simulink model "DataCenterStability"  (R2025b)
settings: Solver=daessc  StartTime=0  StopTime=7  FixedStep=5e-5  MaxStep=0.001  RelTol=1e-3
PostLoadFcn:
  | DataCenterParamScan
InitFcn:
  | opFile_ = fullfile(fileparts(which('DataCenterStability')), 'DataCenterStability_SteadyStateOP.mat');
  | if isfile(opFile_)
  |     tmp_ = load(opFile_, 'op');
  |     assignin('base', 'ssOP__', tmp_.op);
  | end
  | warning('off','physmod:common:mf:system:xform:DelayUnsupportedWithOperatingPoint');
  | warning('off','physmod:common:mf:system:xform:TimeUnsupportedWithOperatingPoint');
values from neighbouring files (symbols this model uses):
  baseVoltageDC = ups.Vdc    [DataCenterParamScan.m]
  bessConverterEfficiency = ups.DCBus.converterEff    [DataCenterParamScan.m]
  droopGain = ups.DCBus.droop    [DataCenterParamScan.m]
  filterInductance = ups.inverter.filterInductance    [DataCenterParamScan.m]
  filterInductanceAFE = ups.AFE.filterInductance    [DataCenterParamScan.m]
  filterResistance = ups.inverter.filterResistance    [DataCenterParamScan.m]
  filterResistanceAFE = ups.AFE.filterResistance    [DataCenterParamScan.m]
  frequency = ups.frequency    [DataCenterParamScan.m]
  G1 = 1    [DataCenterParamScan.m]
  G2 = 0    [DataCenterParamScan.m]
  iBatt = ups.batt.iRated    [DataCenterParamScan.m]
  initialMode = ups.batt.initialMode    [DataCenterParamScan.m]
  invKiId = ups.inverter.kiId    [DataCenterParamScan.m]
  invKiVd = ups.inverter.kiVd    [DataCenterParamScan.m]
  invKpId = ups.inverter.kpId    [DataCenterParamScan.m]
  invKpVd = ups.inverter.kpVd    [DataCenterParamScan.m]
  kpDC = ups.DCBus.kpDC    [DataCenterParamScan.m]
  N_pfc = round(N_total * [1/3, 1/3, 1/3])    [DataCenterParamScan.m]    (also in StabilityStudy.m = cfg.Topology.N_pfc)
  plantRating = ups.rating    [DataCenterParamScan.m]
  powerTau = 0.005    [DataCenterParamScan.m]
  rampRate = ups.batt.rampRate    [DataCenterParamScan.m]
  scan = obj.Cfg.GNC    [GNCAnalyzer.m]
  Ts = 5e-5    (= 5e-05)    [DataCenterParamScan.m]
  Vac = ups.Vac    [DataCenterParamScan.m]
  vBattMax = ups.batt.VMax    [DataCenterParamScan.m]
  vBattNom = ups.batt.Vnom    [DataCenterParamScan.m]
  vDCThreshold = ups.DCBus.VThreshold    [DataCenterParamScan.m]
  vGridMin = ups.DCBus.gridThreshold    [DataCenterParamScan.m]
undefined symbols (not defined in the file or in its folder): ctLimitDelayTime, DiscIntNeverNeededParam, ee_sli_rtmsupport, gcbh, itTray, pfc, serverTray, ups
libraries: fl_lib x77, nesl_utility x35, ee_lib x30, simulink x17, eeGeneralControl x14, datacenter_lib x12, eeTransforms x7, slpidlib x4, nesl_utility_internal x4, simulink_extras x3, datacenterCompositeLib x2, eePowerMeasurement x2
(part 2 of 5)

== system DataCenterStability/IT Load C ==
  " IT Load" : ee_lib/Passive/Dynamic Load  load_type=ee.enum.dc_ac.dc  min_supply_voltage=0.5 V  pow_min=1e-3 W  G_reverse=1e-6 S  deltaV=1e-3 V  f0=60 Hz  Vrms_min=200 V  tau=0.01 s  Vrms_ini=300 V  Vang_ini=0 deg
      settings: InternalSimscapePortConfiguration="{\"Bottom\":[],\"Left\":[{\"id\":\"p\",\"label\":\"+\",\"type\":\"foundation.electrical.electrical\"}],\"Right\":[{\"id\":\"n\",\"label\":\"-\",\"type\":\"foundation.electrical.electrical\"}],\"Top\":[{\"id\":\"P\",\"label\":\"P\",\"type\":\"input\"}]}"
  Capacitor : fl_lib/Electrical/Electrical Elements/Capacitor  c=1e-3 F  r=1e-4 Ohm  g=1e-6 1/Ohm  i_specify=off  i_priority=None  i=0 A  i_nominal_specify=off  i_nominal_value=1  i_nominal_unit=A  v_specify=off  v_priority=None  v=0 V  v_nominal_specify=off  v_nominal_value=1  v_nominal_unit=V  vc_specify=on  vc_priority=Low  vc=400 V  vc_nominal_specify=off  vc_nominal_value=1  vc_nominal_unit=V
  Current Sensor : fl_lib/Electrical/Electrical Sensors/Current Sensor
  DC-DC Converter : ee_lib/Semiconductors & Converters/Converters/DC-DC Converter  Vref_option=ee.enum.converters.voltageref.internal  v_ref=1 V  P_rated=itTray.dcdc.P_rated(3) MW  droop_enabled=false  droop_param=ee.enum.converters.droop.value  droop=0.1 V/A  droop_percent=2  Vref_droop=10 V  reversible=ee.enum.converters.directionality.unidirectional  G_diode=1e-8 1/Ohm  P_fixed=1 W  losses_option=ee.enum.converters.lossesOption.proportionalToSquaredCurrent  eff_rated=itTray.dcdc.eff * 100  tableOption=ee.enum.converters.lossTableOptionThermal.currentTemp  i_eff_vec=[-2, -1, 1, 2] A  v_eff_vec=[15, 30, 45] V  eff_vec=[66, 76, 80, 74]  eff_2D_table=[66, 66, 66; 76, 76, 76; 80, 80, 80; 74, 74, 74]  model_dynamics=ee.enum.converters.dynamics.no  tau=0.02 s  v_ini=10 V  v1_min=1 V  R1=1000 Ohm  R2=1000 Ohm  fault_condition=ee.enum.faults.faultInputCondition.greaterThan  fault_threshold=0.5  T_eff_vec=[280, 300, 320] K  eff_3D_table=repmat([66; 76; 80; 74], 1, 3, 3)  thermal_mass=100 J/K  initial_temperature=298.15 K
      settings: InternalSimscapePortConfiguration="{\"Bottom\":[],\"Left\":[{\"id\":\"p1\",\"label\":\"1+\",\"type\":\"foundation.electrical.electrical\"},{\"id\":\"n1\",\"label\":\"1-\",\"type\":\"foundation.electrical.electrical\"}],\"Right\":[{\"id\":\"p2\",\"label\":\"2+\",\"type\":\"foundation.electrical.electrical\"},{\"id\":\"n2\",\"label\":\"2-\",\"type\":\"foundation.electrical.electrical\"},{\"id\":\"H\",\"label\":\"H\",\"type\":\"foundation.thermal.thermal\"}],\"Top\":[]}"
  Electrical Reference : fl_lib/Electrical/Electrical Elements/Electrical Reference
  PDU Racks : Subsystem  mask{nTrays=36, nRacks=6, trayMass=serverTray.trayMass, trayCp=serverTray.trayCp, trayThermalR=serverTray.trayThermalR_perGPU / itTray.nGPU(3), nGPU=itTray.nGPU(3), gpuTDPperDie=serverTray.gpuTDPperDie, gpuIdlePower=serverTray.gpuIdlePower, gpuHBMpower=serverTray.gpuHBMpower, gpuExponent=serverTray.gpuExponent, gpuHBMutil=serverTray.gpuHBMutil, gpuLeakage=serverTray.gpuLeakage, gpuNominalDieT=serverTray.gpuNominalDieT, gpuDieThermalC=serverTray.gpuDieThermalC_perGPU * itTray.nGPU(3), gpuHeatSinkR=serverTray.gpuHeatSinkR_perGPU / itTray.nGPU(3), gpuSurfArea=serverTray.gpuSurfArea_perGPU * itTray.nGPU(3), gpuAmbientR=serverTray.gpuAmbientR_perGPU / itTray.nGPU(3), nCPU=itTray.nCPU(3), cpuTDPperSocket=350, cpuIdlePower=80, cpuExponent=1.1, cpuLeakage=0.05, cpuNominalDieT=350, cpuDieThermalC=50, cpuHeatSinkR=0.15, cpuSurfArea=0.01, cpuAmbientR=0.5, initialT=serverTray.initialT, htc=serverTray.htc}
      mask prompts: nTrays "Number of IT trays per rack (-)"; nRacks "Number of racks (-)"; trayMass "Tray mass (kg)"; trayCp "Tray specific heat capacity (J/kg*K)"; trayThermalR "Tray to external thermal resistance (K/W)"; nGPU "Number of GPU per tray (-)"; gpuTDPperDie "GPU TDP per die (W)"; gpuIdlePower "GPU idle power (W)"; gpuHBMpower "HBM power per GPU (W)"; gpuExponent "GPU power utilization exponent (-)"; gpuHBMutil "HBM utilization as fraction of compute utilization (-)"; gpuLeakage "Leakage increase per K above nominal temperature (W/K)"; gpuNominalDieT "Nominal die temperature at TDP (K)"; gpuDieThermalC "GPU die thermal capacitance (J/K)"; gpuHeatSinkR "GPU die-heat-sink thermal resistance (K/W)"; gpuSurfArea "Surface area per die for ambient heat transfer (m^2)"; gpuAmbientR "GPU die-ambient thermal resistance (K/W)"; nCPU "Number of CPU per tray (-)"; cpuTDPperSocket "CPU TDP per socket (W)"; cpuIdlePower "CPU idle power per socket (W)"; cpuExponent "CPU power utilization exponent (-)"; cpuLeakage "Leakage increase per K above nominal temperature (W/K)"; cpuNominalDieT "Nominal die temperature at TDP (K)"; cpuDieThermalC "CPU die thermal capacitance (J/K)"; cpuHeatSinkR "CPU die-heat-sink thermal resistance (K/W)"; cpuSurfArea "Surface area per die for ambient heat transfer (m^2)"; cpuAmbientR "CPU die-ambient thermal resistance (K/W)"; initialT "Initial temperature (K)"; htc "Heat transfer coefficient to ambient (W/m^2.K)"
      settings: CopyFcn=set_param(gcbh,'LinkStatus','none');  PortSchema="{\"entries\":[{\"content\":{\"sides\":[{\"content\":{\"connectorIds\":[\"LConn1\",\"LConn2\",\"LConn3\"]},\"type\":\"ConnectorPlacement.EquallySpacedRectSide\",\"uuid\":\"1a9a884a-dab1-4495-bf62-c6b2de6c1039\"},{\"content\":{\"connectorIds\":[\"RConn1\",\"RConn2\",\"RConn3\"],\"side\":\"RIGHT\"},\"type\":\"ConnectorPlacement.EquallySpacedRectSide\",\"uuid\":\"05c53434-51c1-4fee-b885-c321dcda8b6b\"},{\"content\":{\"side\":\"TOP\"},\"type\":\"ConnectorPlacement.EquallySpacedRectSide\",\"uuid\":\"c7b5c534-d596-4858-a133-27f005e6c9d4\"},{\"content\":{\"connectorIds\":[\"RConn4\"],\"side\":\"BOTTOM\"},\"type\":\"ConnectorPlacement.EquallySpacedRectSide\",\"uuid\":\"693f3c99-4296-4d86-bfcc-da753d3e576f\"}]},\"type\":\"ConnectorPlacement.EquallySpacedConnector\",\"uuid\":\"ed91c467-c4d0-403f-af16-bac0257594fd\"}],\"packageUris\":[\"http://schema.mathworks.com/mf0/Connector/R2020b\"],\"version\":\"1.0\"}"
      mask Help: web("DocumentationPDURacks.html")
      mask DialogControl Container10 Prompt: PDU Racks
      mask DialogControl getRatingButton Prompt: Get Rating
      mask DialogControl Container9 Prompt: IT Tray
      mask DialogControl Container6 Prompt: GPU
      mask DialogControl Container7 Prompt: CPU
      mask DialogControl Container8 Prompt: Initial Conditions
      mask Display: image('icon_PDURacks.png');
  PS Gain : fl_lib/Physical Signals/Functions/PS Gain  gain=0.1
  PS Product : fl_lib/Physical Signals/Functions/PS Product
  PS-Simulink Converter : nesl_utility/PS-Simulink Converter  PhysicalDomain=network_engine_domain  SubClassName=ps_output  LeftPortType=input  RightPortType=output  PseudoPeriodic=off  Frequencies=[]  VectorFormat=inherit  Unit=inherit  AffineConversion=off
  PS-Simulink Converter1 : nesl_utility/PS-Simulink Converter  PhysicalDomain=network_engine_domain  SubClassName=ps_output  LeftPortType=input  RightPortType=output  PseudoPeriodic=off  Frequencies=[]  VectorFormat=inherit  Unit=inherit  AffineConversion=off
  PS-Simulink Converter2 : nesl_utility/PS-Simulink Converter  PhysicalDomain=network_engine_domain  SubClassName=ps_output  LeftPortType=input  RightPortType=output  PseudoPeriodic=off  Frequencies=[]  VectorFormat=inherit  Unit=inherit  AffineConversion=off
  Voltage Sensor : fl_lib/Electrical/Electrical Sensors/Voltage Sensor
  - : PMIOPort  Side=Left
  + : PMIOPort  Port=2  Side=Left
  U : PMIOPort  Port=3  Side=Left
  Pe : Outport
  TGPU : Outport  Port=2
  TCPU : Outport  Port=3
  wires:
  PS-Simulink Converter1/1 -> Pe/1
  PS-Simulink Converter/1 -> TGPU/1
  PS-Simulink Converter2/1 -> TCPU/1
  connections:
  DC-DC Converter/RConn1 -- Capacitor/LConn1 -- " IT Load"/LConn1
  -/RConn1 -- DC-DC Converter/LConn2 -- Voltage Sensor/RConn2
  DC-DC Converter/RConn2 -- Electrical Reference/LConn1 -- " IT Load"/RConn1 -- Capacitor/RConn1
  +/RConn1 -- Voltage Sensor/LConn1 -- Current Sensor/LConn1
  PS-Simulink Converter1/LConn1 -- PS Product/RConn1
  Current Sensor/RConn2 -- DC-DC Converter/LConn1
  PS Product/LConn1 -- Voltage Sensor/RConn1
  Current Sensor/RConn1 -- PS Product/LConn2
  PS Gain/LConn1 -- U/RConn1 -- PDU Racks/LConn1
  PS Gain/RConn1 -- PDU Racks/LConn2
  PDU Racks/RConn1 -- " IT Load"/LConn2
  PDU Racks/RConn2 -- PS-Simulink Converter/LConn1
  PDU Racks/RConn3 -- PS-Simulink Converter2/LConn1

== system DataCenterStability/Measurement A ==
  Measurements : Subsystem
  in : PMIOPort  Side=Left
  out : PMIOPort  Port=2  Side=Right
  VRMS : Outport
  wires:
  Measurements/3(VRMS) -> VRMS/1
  connections:
  Measurements/RConn1 -- out/RConn1
  in/RConn1 -- Measurements/LConn1

== system DataCenterStability/Scan Block ==
  AC Scan : Subsystem  ReferencedSubsystem=ScanBlockwithDC  F0=grid.frequency  Theta0=0  Kp_LF=ups.AFE.kpPLL  Ki_LF=ups.AFE.kiPLL  Ts=5e-5  voltage=ups.Vac  voltagedc=ups.Vdc  mva=ups.rating*1e3  Amplitude=scan.Vd  Amplitude1=scan.Vq  Amplitudedc=scan.Vdc  f=scan.f  T=1/scan.samplingfrequency  Tdis=scan.start  Tend=scan.end  VSelect=Equivalent Series Voltage (V)  Hold=Yes
  Constant : Constant  Value=0
  PS-Simulink Converter1 : nesl_utility/PS-Simulink Converter  PhysicalDomain=network_engine_domain  SubClassName=ps_output  LeftPortType=input  RightPortType=output  PseudoPeriodic=off  Frequencies=[]  VectorFormat=inherit  Unit=inherit  AffineConversion=off
  PS-Simulink Converter2 : nesl_utility/PS-Simulink Converter  PhysicalDomain=network_engine_domain  SubClassName=ps_output  LeftPortType=input  RightPortType=output  PseudoPeriodic=off  Frequencies=[]  VectorFormat=inherit  Unit=inherit  AffineConversion=off
  Terminator : Terminator
  To Workspace : ToWorkspace  VariableName=dataAc  SaveFormat=Timeseries  SampleTime=-1
  To Workspace6 : ToWorkspace  VariableName=Idq  SaveFormat=Timeseries  SampleTime=Ts
  To Workspace7 : ToWorkspace  VariableName=Vdq  SaveFormat=Timeseries  SampleTime=Ts
  AC out : PMIOPort  Side=Left
  Iabc : PMIOPort  Port=2  Side=Right
  Vabc : PMIOPort  Port=3  Side=Right
  AC in : PMIOPort  Port=4  Side=Right
  wires:
  PS-Simulink Converter2/1 -> AC Scan/2
  AC Scan/3 -> To Workspace7/1
  AC Scan/2 -> To Workspace6/1
  Constant/1 -> AC Scan/1
  PS-Simulink Converter1/1 -> AC Scan/3
  AC Scan/4 -> Terminator/1
  AC Scan/1 -> To Workspace/1
  connections:
  PS-Simulink Converter1/LConn1 -- Iabc/RConn1
  PS-Simulink Converter2/LConn1 -- Vabc/RConn1
  AC Scan/RConn1 -- AC out/RConn1
  AC Scan/LConn1 -- AC in/RConn1

== system DataCenterStability/UPS ==
  iChrg : Inport
  DC-Link : Subsystem
      settings: CopyFcn=set_param(gcbh,'LinkStatus','none');
      mask Display: image('DCBusbattery_1_1_1.png');
  Inverter : Subsystem
      settings: PortSchema="{\"entries\":[{\"content\":{\"sides\":[{\"content\":{\"connectorIds\":[\"LConn1\",\"Out1\"]},\"type\":\"ConnectorPlacement.EquallySpacedRectSide\",\"uuid\":\"30eca24e-4a0d-4322-ab8d-7623f6b77d91\"},{\"content\":{\"connectorIds\":[\"In1\",\"RConn1\",\"RConn2\"],\"side\":\"RIGHT\"},\"type\":\"ConnectorPlacement.EquallySpacedRectSide\",\"uuid\":\"08a32252-dd7d-4c32-87e9-6b7a03d2f0b7\"},{\"content\":{\"side\":\"TOP\"},\"type\":\"ConnectorPlacement.EquallySpacedRectSide\",\"uuid\":\"b32a0ebb-b906-46f8-8fa8-e8ceac70a0fa\"}]},\"type\":\"ConnectorPlacement.EquallySpacedConnector\",\"uuid\":\"2dde14a6-acee-4d4e-9286-e85271f40ce0\"}],\"packageUris\":[\"http://schema.mathworks.com/mf0/Connector/R2020b\"],\"version\":\"1.0\"}"
      mask Display: image('Copy_2_of_Inverter.png');
  Rectifier : Subsystem
      mask Display: image('rectifier_1_1_1.png');
  ABC : PMIOPort  Side=Left
  ~ : PMIOPort  Port=2  Side=Right
  Meas : Outport
  wires:
  DC-Link/1(Meas) -> Rectifier/1(Meas), Inverter/1(DCMeas)
  Rectifier/1(Id) -> DC-Link/2(iPFC)
  iChrg/1 -> DC-Link/1(iChrg)
  Inverter/1(Meas) -> Meas/1
  Rectifier/2(V) -> DC-Link/3(vPCC)
  Rectifier/3(Brk) -> DC-Link/4(Brk)
  connections:
  Rectifier/RConn2 -- DC-Link/LConn2
  Rectifier/LConn1 -- ABC/RConn1
  Inverter/LConn1 -- ~/RConn1
  DC-Link/RConn1 -- Inverter/RConn1
  Inverter/RConn2 -- DC-Link/RConn2
  DC-Link/LConn1 -- Rectifier/RConn1

== system DataCenterStability/Utility A ==
  V : Inport
  Constant : Constant
  Controlled Voltage Source (Three-Phase) : ee_lib/Sources/Controlled Voltage Source (Three-Phase)  input_option=ee.enum.inputType.singleFreqAC  FRated=60 Hz
      settings: InternalSimscapePortConfiguration="{\"Bottom\":[],\"Left\":[{\"id\":\"Vt\",\"label\":\"Vt\",\"type\":\"input\"},{\"id\":\"ph\",\"label\":\"ph\",\"type\":\"input\"},{\"id\":\"n\",\"label\":\"n\",\"type\":\"foundation.electrical.electrical\"}],\"Right\":[{\"id\":\"N\",\"label\":\"~\",\"type\":\"foundation.electrical.three_phase\"}],\"Top\":[]}"
  Demux : Demux  Outputs=3
  Gain : Gain  Gain=480
  PID Controller : slpidlib/PID Controller  Controller=PI  Form=Parallel  TimeDomain=Discrete-time  UseExternalTs=off  SampleTime=5e-5  IntegratorMethod=Forward Euler  FilterMethod=Forward Euler  ControllerParametersSource=internal  P=1  I=20  UseKiTs=off  D=0  UseExternalDerivativeSource=off  N=100  UseFilter=on  TunerSelectOption=Transfer Function Based (PID Tuner App)  InitialConditionSource=internal  InitialConditionForIntegrator=1  InitialConditionForFilter=0  DifferentiatorICPrevScaledInput=0  ExternalReset=none  TrackingMode=off  Kt=1  LimitOutput=on  SatLimitsSource=internal  UpperSaturationLimit=1.2  LowerSaturationLimit=0.8  LinearizeAsGain=on  AntiWindupMode=clamping  Kb=1  LimitIntegrator=off  UpperIntegratorSaturationLimit=4  LowerIntegratorSaturationLimit=-4  POutMin=[]  POutMax=[]  IOutMin=[]  IOutMax=[]  DOutMin=[]  DOutMax=[]  NOutMin=[]  NOutMax=[]  SumOutMin=[]  SumOutMax=[]  SaturationOutMin=[]  SaturationOutMax=[]  PParamMin=[]  PParamMax=[]  IParamMin=[]  IParamMax=[]  DParamMin=[]  DParamMax=[]  NParamMin=[]  NParamMax=[]  KbParamMin=[]  KbParamMax=[]  KtParamMin=[]  KtParamMax=[]  KbOutMin=[]  KbOutMax=[]  KtOutMin=[]  KtOutMax=[]  IntegratorOutMin=[]  IntegratorOutMax=[]  FilterOutMin=[]  FilterOutMax=[]  SumI1OutMin=[]  SumI1OutMax=[]  SumI2OutMin=[]  SumI2OutMax=[]  SumI3OutMin=[]  SumI3OutMax=[]  SumI4OutMin=[]  SumI4OutMax=[]  SumDOutMin=[]  SumDOutMax=[]  DifferentiatorOutMin=[]  DifferentiatorOutMax=[]  FilterDiffOutCoefMin=[]  FilterDiffOutCoefMax=[]  ReciprocalOutMin=[]  ReciprocalOutMax=[]  SumDenOutMin=[]  SumDenOutMax=[]  SumNumOutMin=[]  SumNumOutMax=[]  DivideOutMin=[]  DivideOutMax=[]  UdiffTsProdOutMin=[]  UdiffTsProdOutMax=[]  NTsProdOutMin=[]  NTsProdOutMax=[]  UintegralTsProdOutMin=[]  UintegralTsProdOutMax=[]  UngainTsProdOutMin=[]  UngainTsProdOutMax=[]  ClampingZeroOutDataTypeStr=Inherit: Inherit via back propagation  ClampingZeroOutMin=[]  ClampingZeroOutMax=[]  FilterDenConstantOutDataTypeStr=Inherit: Inherit via back propagation  FilterDenConstantOutMin=[]  FilterDenConstantOutMax=[]  PCopyOutDataTypeStr=Inherit: Inherit via back propagation  PCopyOutMin=[]  PCopyOutMax=[]  NCopyOutDataTypeStr=Inherit: Inherit via back propagation  NCopyOutMin=[]  NCopyOutMax=[]  IntegratorContinuousStateAttributes=''  IntegratorStateMustResolveToSignalObject=off  IntegratorRTWStateStorageClass=Auto  FilterContinuousStateAttributes=''  FilterStateMustResolveToSignalObject=off  FilterRTWStateStorageClass=Auto  ParallelPVariant=InternalParameters  IdealPVariant=Disabled  IVariant=InternalParameters  DVariant=Disabled  IntegratorVariant=Discrete  SatVariant=Enabled  AWVariant=DiscClampingParallel  PCopyVariant=Disabled  TRVariant=Disabled  FdbkBlocksVariant=Forward  IdealPFdbkVariant=Disabled  SatFdbkVariant=Disabled  DerivativeFilterVariant=Disabled  NVariant=Disabled  NCopyVariant=Disabled_SignalSpec  FilterICVariant=Disabled  IntegratorICVariant=InternalICs  ExternalResetVariant=Disabled  TRSumVariant=Passthrough  SumFdbkVariant=Disabled  SumVariant=Sum_PI  TsampFilterVariant=InternalTs  TsampNgainVariant=Passthrough  TsampIntegralVariant=Disabled_SignalSpec  ExternalSaturationOutDataTypeStr=Inherit: Same as second input  DerivativeSourceVariant=Disabled  PreIntVariant=InternalPreInt
  PS Constant1 : fl_lib/Physical Signals/Sources/PS Constant  constant=0
  Simulink-PS Converter : nesl_utility/Simulink-PS Converter  PhysicalDomain=network_engine_domain  SubClassName=ps_input  LeftPortType=input  RightPortType=output  PseudoPeriodic=off  Frequencies=[]  NoiseDistribution=none  NoiseParameters=[]  Unit=1  AffineConversion=off  FilteringAndDerivatives=filter  SimscapeFilterOrder=1  InputFilterTimeConstant=1e-4  UdotUserProvided=0
  Sum : Sum  Inputs=|-+
  Unit Delay : UnitDelay  InitialCondition=1  SampleTime=5e-5  HasFrameUpgradeWarning=on
  " " : PMIOPort  Side=Left
  " N" : PMIOPort  Port=2  Side=Right
  wires:
  Constant/1 -> Sum/2
  Sum/1 -> PID Controller/1
  PID Controller/1 -> Gain/1
  Gain/1 -> Simulink-PS Converter/1
  V/1 -> Demux/1
  Unit Delay/1 -> Sum/1
  Demux/1 -> Unit Delay/1
  connections:
  " N"/RConn1 -- Controlled Voltage Source (Three-Phase)/LConn3
  Controlled Voltage Source (Three-Phase)/RConn1 -- " "/RConn1
  PS Constant1/RConn1 -- Controlled Voltage Source (Three-Phase)/LConn2
  Controlled Voltage Source (Three-Phase)/LConn1 -- Simulink-PS Converter/RConn1

== system DataCenterStability/CB B/Subsystem1 ==
  input0 : Inport
  Gain : Gain  Gain=1e9
  Phase Splitter : ee_lib/Connectors & References/Phase Splitter
  Phase Splitter1 : ee_lib/Connectors & References/Phase Splitter
  Simulink-PS Converter : nesl_utility/Simulink-PS Converter  PhysicalDomain=network_engine_domain  SubClassName=ps_input  LeftPortType=input  RightPortType=output  PseudoPeriodic=off  Frequencies=[]  NoiseDistribution=none  NoiseParameters=[]  Unit=1  AffineConversion=off  FilteringAndDerivatives=provide  SimscapeFilterOrder=1  InputFilterTimeConstant=0.001  UdotUserProvided=0
  Variable Resistor : fl_lib/Electrical/Electrical Elements/Variable Resistor  Rmin=1e-4 Ohm  thermalEnable=false  thermal_mass=1 J/K  i_specify=off  i_priority=None  i=0 A  i_nominal_specify=off  i_nominal_value=1  i_nominal_unit=A  v_specify=off  v_priority=None  v=0 V  v_nominal_specify=off  v_nominal_value=1  v_nominal_unit=V  T_specify=off  T_priority=None  T=300 K  T_nominal_specify=off  T_nominal_value=1  T_nominal_unit=K
  Variable Resistor1 : fl_lib/Electrical/Electrical Elements/Variable Resistor  Rmin=1e-4 Ohm  thermalEnable=false  thermal_mass=1 J/K  i_specify=off  i_priority=None  i=0 A  i_nominal_specify=off  i_nominal_value=1  i_nominal_unit=A  v_specify=off  v_priority=None  v=0 V  v_nominal_specify=off  v_nominal_value=1  v_nominal_unit=V  T_specify=off  T_priority=None  T=300 K  T_nominal_specify=off  T_nominal_value=1  T_nominal_unit=K
  Variable Resistor2 : fl_lib/Electrical/Electrical Elements/Variable Resistor  Rmin=1e-4 Ohm  thermalEnable=false  thermal_mass=1 J/K  i_specify=off  i_priority=None  i=0 A  i_nominal_specify=off  i_nominal_value=1  i_nominal_unit=A  v_specify=off  v_priority=None  v=0 V  v_nominal_specify=off  v_nominal_value=1  v_nominal_unit=V  T_specify=off  T_priority=None  T=300 K  T_nominal_specify=off  T_nominal_value=1  T_nominal_unit=K
  Conn1 : PMIOPort  Side=Left
  Conn2 : PMIOPort  Port=2  Side=Right
  wires:
  input0/1 -> Gain/1
  Gain/1 -> Simulink-PS Converter/1
  connections:
  Variable Resistor2/LConn1 -- Variable Resistor1/LConn1 -- Simulink-PS Converter/RConn1 -- Variable Resistor/LConn1
  Phase Splitter/LConn1 -- Conn2/RConn1
  Phase Splitter/RConn1 -- Variable Resistor/LConn2
  Phase Splitter/RConn2 -- Variable Resistor1/LConn2
  Phase Splitter/RConn3 -- Variable Resistor2/LConn2
  Phase Splitter1/LConn1 -- Conn1/RConn1
  Variable Resistor/RConn1 -- Phase Splitter1/RConn1
  Phase Splitter1/RConn2 -- Variable Resistor1/RConn1
  Variable Resistor2/RConn1 -- Phase Splitter1/RConn3

== system DataCenterStability/CB B2/Subsystem1 ==
  input0 : Inport
  Gain : Gain  Gain=1e9
  Phase Splitter : ee_lib/Connectors & References/Phase Splitter
  Phase Splitter1 : ee_lib/Connectors & References/Phase Splitter
  Simulink-PS Converter : nesl_utility/Simulink-PS Converter  PhysicalDomain=network_engine_domain  SubClassName=ps_input  LeftPortType=input  RightPortType=output  PseudoPeriodic=off  Frequencies=[]  NoiseDistribution=none  NoiseParameters=[]  Unit=1  AffineConversion=off  FilteringAndDerivatives=provide  SimscapeFilterOrder=1  InputFilterTimeConstant=0.001  UdotUserProvided=0
  Variable Resistor : fl_lib/Electrical/Electrical Elements/Variable Resistor  Rmin=1e-4 Ohm  thermalEnable=false  thermal_mass=1 J/K  i_specify=off  i_priority=None  i=0 A  i_nominal_specify=off  i_nominal_value=1  i_nominal_unit=A  v_specify=off  v_priority=None  v=0 V  v_nominal_specify=off  v_nominal_value=1  v_nominal_unit=V  T_specify=off  T_priority=None  T=300 K  T_nominal_specify=off  T_nominal_value=1  T_nominal_unit=K
  Variable Resistor1 : fl_lib/Electrical/Electrical Elements/Variable Resistor  Rmin=1e-4 Ohm  thermalEnable=false  thermal_mass=1 J/K  i_specify=off  i_priority=None  i=0 A  i_nominal_specify=off  i_nominal_value=1  i_nominal_unit=A  v_specify=off  v_priority=None  v=0 V  v_nominal_specify=off  v_nominal_value=1  v_nominal_unit=V  T_specify=off  T_priority=None  T=300 K  T_nominal_specify=off  T_nominal_value=1  T_nominal_unit=K
  Variable Resistor2 : fl_lib/Electrical/Electrical Elements/Variable Resistor  Rmin=1e-4 Ohm  thermalEnable=false  thermal_mass=1 J/K  i_specify=off  i_priority=None  i=0 A  i_nominal_specify=off  i_nominal_value=1  i_nominal_unit=A  v_specify=off  v_priority=None  v=0 V  v_nominal_specify=off  v_nominal_value=1  v_nominal_unit=V  T_specify=off  T_priority=None  T=300 K  T_nominal_specify=off  T_nominal_value=1  T_nominal_unit=K
  Conn1 : PMIOPort  Side=Left
  Conn2 : PMIOPort  Port=2  Side=Right
  wires:
  input0/1 -> Gain/1
  Gain/1 -> Simulink-PS Converter/1
  connections:
  Variable Resistor2/LConn1 -- Variable Resistor1/LConn1 -- Simulink-PS Converter/RConn1 -- Variable Resistor/LConn1
  Phase Splitter/LConn1 -- Conn2/RConn1
  Phase Splitter/RConn1 -- Variable Resistor/LConn2
  Phase Splitter/RConn2 -- Variable Resistor1/LConn2
  Phase Splitter/RConn3 -- Variable Resistor2/LConn2
  Phase Splitter1/LConn1 -- Conn1/RConn1
  Variable Resistor/RConn1 -- Phase Splitter1/RConn1
  Phase Splitter1/RConn2 -- Variable Resistor1/RConn1
  Variable Resistor2/RConn1 -- Phase Splitter1/RConn3

== system DataCenterStability/CB B3/Subsystem1 ==
  input0 : Inport
  Gain : Gain  Gain=1e9
  Phase Splitter : ee_lib/Connectors & References/Phase Splitter
  Phase Splitter1 : ee_lib/Connectors & References/Phase Splitter
  Simulink-PS Converter : nesl_utility/Simulink-PS Converter  PhysicalDomain=network_engine_domain  SubClassName=ps_input  LeftPortType=input  RightPortType=output  PseudoPeriodic=off  Frequencies=[]  NoiseDistribution=none  NoiseParameters=[]  Unit=1  AffineConversion=off  FilteringAndDerivatives=provide  SimscapeFilterOrder=1  InputFilterTimeConstant=0.001  UdotUserProvided=0
  Variable Resistor : fl_lib/Electrical/Electrical Elements/Variable Resistor  Rmin=1e-4 Ohm  thermalEnable=false  thermal_mass=1 J/K  i_specify=off  i_priority=None  i=0 A  i_nominal_specify=off  i_nominal_value=1  i_nominal_unit=A  v_specify=off  v_priority=None  v=0 V  v_nominal_specify=off  v_nominal_value=1  v_nominal_unit=V  T_specify=off  T_priority=None  T=300 K  T_nominal_specify=off  T_nominal_value=1  T_nominal_unit=K
  Variable Resistor1 : fl_lib/Electrical/Electrical Elements/Variable Resistor  Rmin=1e-4 Ohm  thermalEnable=false  thermal_mass=1 J/K  i_specify=off  i_priority=None  i=0 A  i_nominal_specify=off  i_nominal_value=1  i_nominal_unit=A  v_specify=off  v_priority=None  v=0 V  v_nominal_specify=off  v_nominal_value=1  v_nominal_unit=V  T_specify=off  T_priority=None  T=300 K  T_nominal_specify=off  T_nominal_value=1  T_nominal_unit=K
  Variable Resistor2 : fl_lib/Electrical/Electrical Elements/Variable Resistor  Rmin=1e-4 Ohm  thermalEnable=false  thermal_mass=1 J/K  i_specify=off  i_priority=None  i=0 A  i_nominal_specify=off  i_nominal_value=1  i_nominal_unit=A  v_specify=off  v_priority=None  v=0 V  v_nominal_specify=off  v_nominal_value=1  v_nominal_unit=V  T_specify=off  T_priority=None  T=300 K  T_nominal_specify=off  T_nominal_value=1  T_nominal_unit=K
  Conn1 : PMIOPort  Side=Left
  Conn2 : PMIOPort  Port=2  Side=Right
  wires:
  input0/1 -> Gain/1
  Gain/1 -> Simulink-PS Converter/1
  connections:
  Variable Resistor2/LConn1 -- Variable Resistor1/LConn1 -- Simulink-PS Converter/RConn1 -- Variable Resistor/LConn1
  Phase Splitter/LConn1 -- Conn2/RConn1
  Phase Splitter/RConn1 -- Variable Resistor/LConn2
  Phase Splitter/RConn2 -- Variable Resistor1/LConn2
  Phase Splitter/RConn3 -- Variable Resistor2/LConn2
  Phase Splitter1/LConn1 -- Conn1/RConn1
  Variable Resistor/RConn1 -- Phase Splitter1/RConn1
  Phase Splitter1/RConn2 -- Variable Resistor1/RConn1
  Variable Resistor2/RConn1 -- Phase Splitter1/RConn3

== system DataCenterStability/IT  Load A/PDU Racks ==
  PS Product : fl_lib/Physical Signals/Functions/PS Product
  Server Tray : Subsystem  mask{nGPU=nGPU, gpuTDPperDie=gpuTDPperDie, gpuIdlePower=gpuIdlePower, gpuHBMpower=gpuHBMpower, gpuExponent=gpuExponent, gpuHBMutil=gpuHBMutil, gpuLeakage=gpuLeakage, gpuNominalDieT=gpuLeakage, gpuDieThermalC=gpuDieThermalC, gpuHeatSinkR=gpuHeatSinkR, gpuSurfArea=gpuSurfArea, gpuAmbientR=gpuAmbientR, nCPU=nCPU, cpuTDPperSocket=cpuTDPperSocket, cpuIdlePower=cpuIdlePower, cpuExponent=cpuExponent, cpuLeakage=cpuLeakage, cpuNominalDieT=cpuNominalDieT, cpuDieThermalC=cpuDieThermalC, cpuHeatSinkR=cpuHeatSinkR, cpuSurfArea=cpuSurfArea, cpuAmbientR=cpuAmbientR, trayMass=trayMass, trayCp=trayCp, trayThermalR=trayThermalR, initialT=initialT, htc=htc}
      mask prompts: nGPU "Number of GPU (-)"; gpuTDPperDie "GPU TDP per die (W)"; gpuIdlePower "GPU idle power (W)"; gpuHBMpower "HBM power per GPU (W)"; gpuExponent "GPU power utilization exponent (-)"; gpuHBMutil "HBM utilization as fraction of compute utilization (-)"; gpuLeakage "Leakage increase per K above nominal temperature (W/K)"; gpuNominalDieT "Nominal die temperature at TDP (K)"; gpuDieThermalC "GPU die thermal capacitance (J/K)"; gpuHeatSinkR "GPU die-heat-sink thermal resistance (K/W)"; gpuSurfArea "Surface area per die for ambient heat transfer (m^2)"; gpuAmbientR "GPU die-ambient thermal resistance (K/W)"; nCPU "Number of CPU (-)"; cpuTDPperSocket "CPU TDP per socket (W)"; cpuIdlePower "CPU idle power per socket (W)"; cpuExponent "CPU power utilization exponent (-)"; cpuLeakage "Leakage increase per K above nominal temperature (W/K)"; cpuNominalDieT "Nominal die temperature at TDP (K)"; cpuDieThermalC "CPU die thermal capacitance (J/K)"; cpuHeatSinkR "CPU die-heat-sink thermal resistance (K/W)"; cpuSurfArea "Surface area per die for ambient heat transfer (m^2)"; cpuAmbientR "CPU die-ambient thermal resistance (K/W)"; trayMass "Tray mass (kg)"; trayCp "Tray specific heat capacity (J/kg*K)"; trayThermalR "Tray to external thermal resistance (K/W)"; initialT "Initial temperature (K)"; htc "Heat transfer coefficient to ambient (W/m^2.K)"
      settings: CopyFcn=set_param(gcbh,'LinkStatus','none');  PortSchema="{\"entries\":[{\"content\":{\"sides\":[{\"content\":{\"connectorIds\":[\"LConn1\",\"LConn2\",\"LConn3\"]},\"type\":\"ConnectorPlacement.EquallySpacedRectSide\",\"uuid\":\"893f21b9-92d6-433a-96e5-f8193a696c29\"},{\"content\":{\"connectorIds\":[\"RConn1\",\"RConn2\",\"RConn3\"],\"side\":\"RIGHT\"},\"type\":\"ConnectorPlacement.EquallySpacedRectSide\",\"uuid\":\"efd10409-70d8-4a6a-97a2-13f0e6f538e3\"},{\"content\":{\"side\":\"TOP\"},\"type\":\"ConnectorPlacement.EquallySpacedRectSide\",\"uuid\":\"8c9765cd-90e6-46de-916c-606bbb93143e\"},{\"content\":{\"connectorIds\":[\"RConn4\"],\"side\":\"BOTTOM\"},\"type\":\"ConnectorPlacement.EquallySpacedRectSide\",\"uuid\":\"9656b44e-d582-43b0-a7fe-c629821d6c27\"}]},\"type\":\"ConnectorPlacement.EquallySpacedConnector\",\"uuid\":\"add7a682-eb4b-4f46-a5b9-e161ccf96de5\"}],\"packageUris\":[\"http://schema.mathworks.com/mf0/Connector/R2020b\"],\"version\":\"1.0\"}"
      mask Help: web("DocumentationServerTray.html")
      mask DialogControl Container6 Prompt: GPU
      mask DialogControl Container7 Prompt: CPU
      mask DialogControl Container9 Prompt: IT Tray
      mask DialogControl Container8 Prompt: Initial Conditions
      mask Display: image('icon_serverPlate.png');
  TMamb : datacenter_lib/Thermal Multiplier
      settings: InternalSimscapePortConfiguration="{\"Bottom\":[],\"Left\":[{\"id\":\"A\",\"label\":\"A\",\"type\":\"foundation.thermal.thermal\"}],\"Right\":[{\"id\":\"B\",\"label\":\"B\",\"type\":\"foundation.thermal.thermal\"}],\"Top\":[{\"id\":\"Na\",\"label\":\"Na\",\"type\":\"input\"},{\"id\":\"Nb\",\"label\":\"Nb\",\"type\":\"input\"}]}"
  TMcdu : datacenter_lib/Thermal Multiplier
      settings: InternalSimscapePortConfiguration="{\"Bottom\":[],\"Left\":[{\"id\":\"A\",\"label\":\"A\",\"type\":\"foundation.thermal.thermal\"}],\"Right\":[{\"id\":\"B\",\"label\":\"B\",\"type\":\"foundation.thermal.thermal\"}],\"Top\":[{\"id\":\"Na\",\"label\":\"Na\",\"type\":\"input\"},{\"id\":\"Nb\",\"label\":\"Nb\",\"type\":\"input\"}]}"
  nTraysXnRacks : fl_lib/Physical Signals/Sources/PS Constant  constant=nTrays*nRacks
  one : fl_lib/Physical Signals/Sources/PS Constant  constant=1
  U_gpu : PMIOPort  Side=Left
  U_cpu : PMIOPort  Port=2  Side=Left
  Ha : PMIOPort  Port=3  Side=Left
  P : PMIOPort  Port=4  Side=Right
  T_gpu : PMIOPort  Port=5  Side=Right
  T_cpu : PMIOPort  Port=6  Side=Right
  Hc : PMIOPort  Port=7  Side=Right
  connections:
  Server Tray/LConn1 -- U_gpu/RConn1
  TMamb/LConn1 -- Ha/RConn1
  Server Tray/RConn2 -- T_gpu/RConn1
  TMcdu/RConn1 -- Hc/RConn1
  Server Tray/LConn2 -- U_cpu/RConn1
  Server Tray/RConn3 -- T_cpu/RConn1
  one/RConn1 -- TMcdu/LConn3 -- TMamb/LConn2
  Server Tray/RConn4 -- TMcdu/LConn1
  Server Tray/LConn3 -- TMamb/RConn1
  nTraysXnRacks/RConn1 -- PS Product/LConn1 -- TMcdu/LConn2 -- TMamb/LConn3
  Server Tray/RConn1 -- PS Product/LConn2
  PS Product/RConn1 -- P/RConn1

== system DataCenterStability/IT Load B/PDU Racks ==
  PS Product : fl_lib/Physical Signals/Functions/PS Product
  Server Tray : datacenterCompositeLib/Server Tray  nGPU=nGPU  gpuTDPperDie=gpuTDPperDie  gpuIdlePower=gpuIdlePower  gpuHBMpower=gpuHBMpower  gpuExponent=gpuExponent  gpuHBMutil=gpuHBMutil  gpuLeakage=gpuLeakage  gpuNominalDieT=gpuLeakage  gpuDieThermalC=gpuDieThermalC  gpuHeatSinkR=gpuHeatSinkR  gpuSurfArea=gpuSurfArea  gpuAmbientR=gpuAmbientR  nCPU=nCPU  cpuTDPperSocket=cpuTDPperSocket  cpuIdlePower=cpuIdlePower  cpuExponent=cpuExponent  cpuLeakage=cpuLeakage  cpuNominalDieT=cpuNominalDieT  cpuDieThermalC=cpuDieThermalC  cpuHeatSinkR=cpuHeatSinkR  cpuSurfArea=cpuSurfArea  cpuAmbientR=cpuAmbientR  trayMass=trayMass  trayCp=trayCp  trayThermalR=trayThermalR  initialT=initialT  htc=htc
  TMamb : datacenter_lib/Thermal Multiplier
      settings: InternalSimscapePortConfiguration="{\"Bottom\":[],\"Left\":[{\"id\":\"A\",\"label\":\"A\",\"type\":\"foundation.thermal.thermal\"}],\"Right\":[{\"id\":\"B\",\"label\":\"B\",\"type\":\"foundation.thermal.thermal\"}],\"Top\":[{\"id\":\"Na\",\"label\":\"Na\",\"type\":\"input\"},{\"id\":\"Nb\",\"label\":\"Nb\",\"type\":\"input\"}]}"
  TMcdu : datacenter_lib/Thermal Multiplier
      settings: InternalSimscapePortConfiguration="{\"Bottom\":[],\"Left\":[{\"id\":\"A\",\"label\":\"A\",\"type\":\"foundation.thermal.thermal\"}],\"Right\":[{\"id\":\"B\",\"label\":\"B\",\"type\":\"foundation.thermal.thermal\"}],\"Top\":[{\"id\":\"Na\",\"label\":\"Na\",\"type\":\"input\"},{\"id\":\"Nb\",\"label\":\"Nb\",\"type\":\"input\"}]}"
  nTraysXnRacks : fl_lib/Physical Signals/Sources/PS Constant  constant=nTrays*nRacks
  one : fl_lib/Physical Signals/Sources/PS Constant  constant=1
  U_gpu : PMIOPort  Side=Left
  U_cpu : PMIOPort  Port=2  Side=Left
  Ha : PMIOPort  Port=3  Side=Left
  P : PMIOPort  Port=4  Side=Right
  T_gpu : PMIOPort  Port=5  Side=Right
  T_cpu : PMIOPort  Port=6  Side=Right
  Hc : PMIOPort  Port=7  Side=Right
  connections:
  PS Product/RConn1 -- P/RConn1
  Server Tray/RConn1 -- PS Product/LConn2
  TMamb/LConn3 -- TMcdu/LConn2 -- PS Product/LConn1 -- nTraysXnRacks/RConn1
  Server Tray/LConn3 -- TMamb/RConn1
  Server Tray/RConn4 -- TMcdu/LConn1
  TMamb/LConn2 -- TMcdu/LConn3 -- one/RConn1
  Server Tray/RConn3 -- T_cpu/RConn1
  Server Tray/LConn2 -- U_cpu/RConn1
  TMcdu/RConn1 -- Hc/RConn1
  Server Tray/RConn2 -- T_gpu/RConn1
  TMamb/LConn1 -- Ha/RConn1
  Server Tray/LConn1 -- U_gpu/RConn1

== system DataCenterStability/IT Load C/PDU Racks ==
  PS Product : fl_lib/Physical Signals/Functions/PS Product
  Server Tray : datacenterCompositeLib/Server Tray  nGPU=nGPU  gpuTDPperDie=gpuTDPperDie  gpuIdlePower=gpuIdlePower  gpuHBMpower=gpuHBMpower  gpuExponent=gpuExponent  gpuHBMutil=gpuHBMutil  gpuLeakage=gpuLeakage  gpuNominalDieT=gpuLeakage  gpuDieThermalC=gpuDieThermalC  gpuHeatSinkR=gpuHeatSinkR  gpuSurfArea=gpuSurfArea  gpuAmbientR=gpuAmbientR  nCPU=nCPU  cpuTDPperSocket=cpuTDPperSocket  cpuIdlePower=cpuIdlePower  cpuExponent=cpuExponent  cpuLeakage=cpuLeakage  cpuNominalDieT=cpuNominalDieT  cpuDieThermalC=cpuDieThermalC  cpuHeatSinkR=cpuHeatSinkR  cpuSurfArea=cpuSurfArea  cpuAmbientR=cpuAmbientR  trayMass=trayMass  trayCp=trayCp  trayThermalR=trayThermalR  initialT=initialT  htc=htc
  TMamb : datacenter_lib/Thermal Multiplier
      settings: InternalSimscapePortConfiguration="{\"Bottom\":[],\"Left\":[{\"id\":\"A\",\"label\":\"A\",\"type\":\"foundation.thermal.thermal\"}],\"Right\":[{\"id\":\"B\",\"label\":\"B\",\"type\":\"foundation.thermal.thermal\"}],\"Top\":[{\"id\":\"Na\",\"label\":\"Na\",\"type\":\"input\"},{\"id\":\"Nb\",\"label\":\"Nb\",\"type\":\"input\"}]}"
  TMcdu : datacenter_lib/Thermal Multiplier
      settings: InternalSimscapePortConfiguration="{\"Bottom\":[],\"Left\":[{\"id\":\"A\",\"label\":\"A\",\"type\":\"foundation.thermal.thermal\"}],\"Right\":[{\"id\":\"B\",\"label\":\"B\",\"type\":\"foundation.thermal.thermal\"}],\"Top\":[{\"id\":\"Na\",\"label\":\"Na\",\"type\":\"input\"},{\"id\":\"Nb\",\"label\":\"Nb\",\"type\":\"input\"}]}"
  nTraysXnRacks : fl_lib/Physical Signals/Sources/PS Constant  constant=nTrays*nRacks
  one : fl_lib/Physical Signals/Sources/PS Constant  constant=1
  U_gpu : PMIOPort  Side=Left
  U_cpu : PMIOPort  Port=2  Side=Left
  Ha : PMIOPort  Port=3  Side=Left
  P : PMIOPort  Port=4  Side=Right
  T_gpu : PMIOPort  Port=5  Side=Right
  T_cpu : PMIOPort  Port=6  Side=Right
  Hc : PMIOPort  Port=7  Side=Right
  connections:
  PS Product/RConn1 -- P/RConn1
  Server Tray/RConn1 -- PS Product/LConn2
  TMamb/LConn3 -- TMcdu/LConn2 -- PS Product/LConn1 -- nTraysXnRacks/RConn1
  Server Tray/LConn3 -- TMamb/RConn1
  Server Tray/RConn4 -- TMcdu/LConn1
  TMamb/LConn2 -- TMcdu/LConn3 -- one/RConn1
  Server Tray/RConn3 -- T_cpu/RConn1
  Server Tray/LConn2 -- U_cpu/RConn1
  TMcdu/RConn1 -- Hc/RConn1
  Server Tray/RConn2 -- T_gpu/RConn1
  TMamb/LConn1 -- Ha/RConn1
  Server Tray/LConn1 -- U_gpu/RConn1

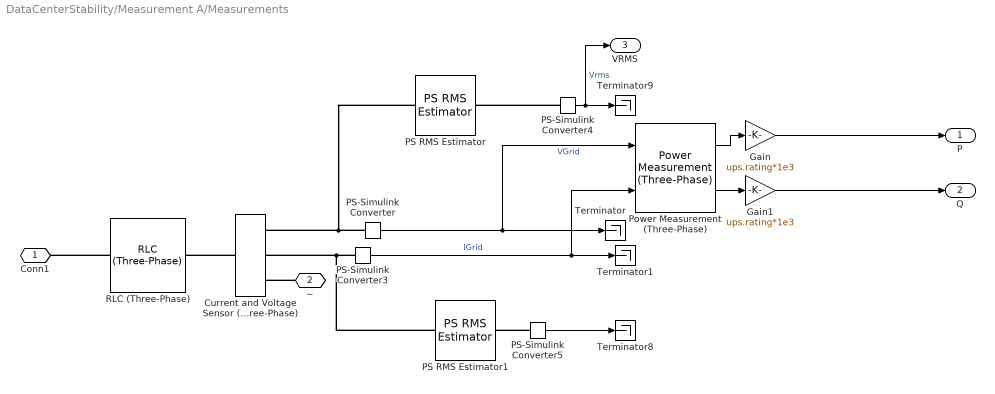
== system DataCenterStability/Measurement A/Measurements ==
  Current and Voltage Sensor (Three-Phase) : ee_lib/Sensors & Transducers/Current and Voltage Sensor (Three-Phase)  vMeasurementType=ee.enum.vmeasurement.ll  outputUnit=ee.enum.unit.pu  SRated=ups.rating*1e3 A*V  VRated=ups.Vac/sqrt(2) V  I_specify=off  I_priority=None  I=[0, 0, 0] A  I_nominal_specify=off  I_nominal_value=1  I_nominal_unit=A  V_specify=off  V_priority=None  V=[0, 0, 0] V  V_nominal_specify=off  V_nominal_value=1  V_nominal_unit=V
      settings: InternalSimscapePortConfiguration="{\"Bottom\":[],\"Left\":[{\"id\":\"N1\",\"label\":\"~1\",\"type\":\"foundation.electrical.three_phase\"}],\"Right\":[{\"id\":\"V_output\",\"label\":\"V\",\"type\":\"output\"},{\"id\":\"I_output\",\"label\":\"I\",\"type\":\"output\"},{\"id\":\"N2\",\"label\":\"~2\",\"type\":\"foundation.electrical.three_phase\"}],\"Top\":[]}"
  Gain : Gain  Gain=ups.rating*1e3
  Gain1 : Gain  Gain=ups.rating*1e3
  PS RMS Estimator : fl_lib/Physical Signals/Periodic Operators/PS RMS Estimator  f0=60 Hz
      settings: InternalSimscapePortConfiguration="{\"Bottom\":[],\"Left\":[{\"id\":\"I\",\"label\":\"\",\"type\":\"input\"}],\"Right\":[{\"id\":\"O\",\"label\":\"\",\"type\":\"output\"}],\"Top\":[]}"
  PS RMS Estimator1 : fl_lib/Physical Signals/Periodic Operators/PS RMS Estimator  f0=60 Hz
      settings: InternalSimscapePortConfiguration="{\"Bottom\":[],\"Left\":[{\"id\":\"I\",\"label\":\"\",\"type\":\"input\"}],\"Right\":[{\"id\":\"O\",\"label\":\"\",\"type\":\"output\"}],\"Top\":[]}"
  PS-Simulink Converter{,3..5} (4 alike) : nesl_utility/PS-Simulink Converter  PhysicalDomain=network_engine_domain  SubClassName=ps_output  LeftPortType=input  RightPortType=output  PseudoPeriodic=off  Frequencies=[]  VectorFormat=inherit  Unit=inherit  AffineConversion=off
  Power Measurement (Three-Phase) : eePowerMeasurement/Power Measurement (Three-Phase)  LabelModeActiveChoice=Discrete  F=60  K=1  Seq=Positive  Ts=Ts
  RLC (Three-Phase) : ee_lib/Passive/RLC Assemblies/RLC (Three-Phase)  port_option=ee.enum.threePhasePort.composite  component_structure=ee.enum.rlc.structure.SeriesRL  R=0.0001 Ohm  L=1e-07 H  C=1e-6 F  R_parasitic=0 Ohm  G_parasitic=0 1/Ohm  IL_specify=on  IL_priority=None  IL=[0, 0, 0] A  IL_nominal_specify=off  IL_nominal_value=1  IL_nominal_unit=A  VC_specify=off  VC_priority=High  VC=[0, 0, 0] V  VC_nominal_specify=off  VC_nominal_value=1  VC_nominal_unit=V
      settings: InternalSimscapePortConfiguration="{\"Bottom\":[],\"Left\":[{\"id\":\"N1\",\"label\":\"~1\",\"type\":\"foundation.electrical.three_phase\"}],\"Right\":[{\"id\":\"N2\",\"label\":\"~2\",\"type\":\"foundation.electrical.three_phase\"}],\"Top\":[]}"
  Terminator{,1,8..9} (4 alike) : Terminator
  Conn1 : PMIOPort  Side=Left
  ~ : PMIOPort  Port=2  Side=Right
  P : Outport
  Q : Outport  Port=2
  VRMS : Outport  Port=3
  wires:
  Gain/1 -> P/1
  PS-Simulink Converter5/1 -> Terminator8/1
  PS-Simulink Converter4/1 -> VRMS/1, Terminator9/1  "Vrms"
  Gain1/1 -> Q/1
  PS-Simulink Converter3/1 -> Power Measurement (Three-Phase)/2, Terminator1/1  "IGrid"
  PS-Simulink Converter/1 -> Power Measurement (Three-Phase)/1, Terminator/1  "VGrid"
  Power Measurement (Three-Phase)/2 -> Gain1/1
  Power Measurement (Three-Phase)/1 -> Gain/1
  connections:
  PS-Simulink Converter3/LConn1 -- Current and Voltage Sensor (Three-Phase)/RConn2 -- PS RMS Estimator1/LConn1
  PS-Simulink Converter/LConn1 -- Current and Voltage Sensor (Three-Phase)/RConn1 -- PS RMS Estimator/LConn1
  ~/RConn1 -- Current and Voltage Sensor (Three-Phase)/RConn3
  PS-Simulink Converter5/LConn1 -- PS RMS Estimator1/RConn1
  Current and Voltage Sensor (Three-Phase)/LConn1 -- RLC (Three-Phase)/RConn1
  PS-Simulink Converter4/LConn1 -- PS RMS Estimator/RConn1
  RLC (Three-Phase)/LConn1 -- Conn1/RConn1

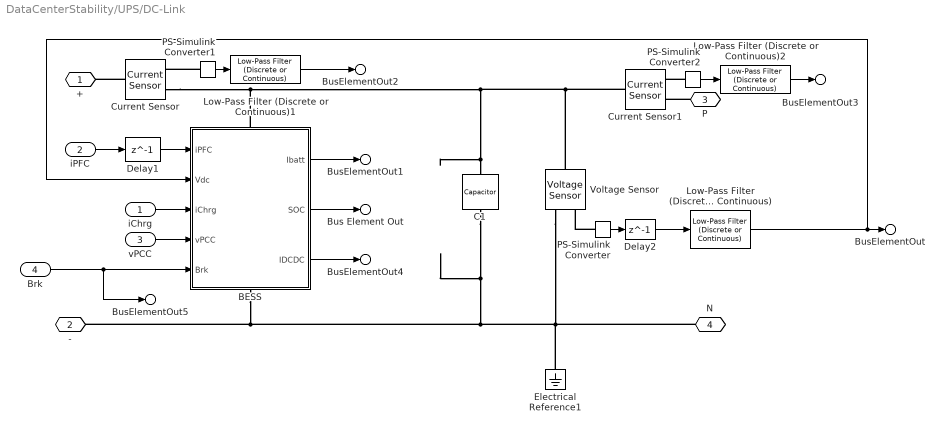
== system DataCenterStability/UPS/DC-Link ==
  iChrg : Inport
  iPFC : Inport  Port=2
  vPCC : Inport  Port=3
  Brk : Inport  Port=4
  BESS : Subsystem
      settings: PortSchema="{\"entries\":[{\"content\":{\"sides\":[{\"content\":{\"connectorIds\":[\"LConn1\"]},\"type\":\"ConnectorPlacement.EquallySpacedRectSide\",\"uuid\":\"dc16109c-3681-46df-aa2d-40033a424f4f\"},{\"content\":{\"connectorIds\":[\"RConn1\"],\"side\":\"RIGHT\"},\"type\":\"ConnectorPlacement.EquallySpacedRectSide\",\"uuid\":\"5490aea4-59f2-45ea-9bac-3971cd260353\"},{\"content\":{\"connectorIds\":[\"Out1\",\"Out2\",\"Out3\"],\"side\":\"TOP\"},\"type\":\"ConnectorPlacement.EquallySpacedRectSide\",\"uuid\":\"92b5185c-680a-4a4f-a590-9680bdd408ad\"},{\"content\":{\"connectorIds\":[\"In1\",\"In2\",\"In3\",\"In4\",\"In5\"],\"side\":\"BOTTOM\"},\"type\":\"ConnectorPlacement.EquallySpacedRectSide\",\"uuid\":\"bb2f2b82-1e61-49ed-8567-aad9343e236f\"}]},\"type\":\"ConnectorPlacement.EquallySpacedConnector\",\"uuid\":\"c23d7033-d24f-41ec-a8dd-f02fcfba4177\"}],\"packageUris\":[\"http://schema.mathworks.com/mf0/Connector/R2020b\"],\"version\":\"1.0\"}"
  C1 : fl_lib/Electrical/Electrical Elements/Capacitor  c=1.6 F  r=1e-3 Ohm  g=0 1/Ohm  i_specify=on  i_priority=None  i=0 A  i_nominal_specify=off  i_nominal_value=1  i_nominal_unit=A  v_specify=off  v_priority=High  v=800 V  v_nominal_specify=off  v_nominal_value=1  v_nominal_unit=V  vc_specify=on  vc_priority=Low  vc=baseVoltageDC V  vc_nominal_specify=off  vc_nominal_value=1  vc_nominal_unit=V
  Current Sensor : fl_lib/Electrical/Electrical Sensors/Current Sensor
  Current Sensor1 : fl_lib/Electrical/Electrical Sensors/Current Sensor
  Delay1 : Delay  DelayLength=1  InitialCondition=1
  Delay2 : Delay  DelayLength=1  InitialCondition=baseVoltageDC
  Electrical Reference1 : fl_lib/Electrical/Electrical Elements/Electrical Reference
  Low-Pass Filter (Discrete or Continuous) : eeGeneralControl/Low-Pass Filter (Discrete or Continuous)  K=1  T=0.001  B=inf  A=-inf  init_option=Inherited from block input  x0=0  Ts=-1
  Low-Pass Filter (Discrete or Continuous)1 : eeGeneralControl/Low-Pass Filter (Discrete or Continuous)  K=1  T=0.001  B=inf  A=-inf  init_option=Inherited from block input  x0=0  Ts=-1
  Low-Pass Filter (Discrete or Continuous)2 : eeGeneralControl/Low-Pass Filter (Discrete or Continuous)  K=1  T=0.001  B=inf  A=-inf  init_option=Inherited from block input  x0=0  Ts=-1
  PS-Simulink Converter : nesl_utility/PS-Simulink Converter  PhysicalDomain=network_engine_domain  SubClassName=ps_output  LeftPortType=input  RightPortType=output  PseudoPeriodic=off  Frequencies=[]  VectorFormat=inherit  Unit=inherit  AffineConversion=off
  PS-Simulink Converter1 : nesl_utility/PS-Simulink Converter  PhysicalDomain=network_engine_domain  SubClassName=ps_output  LeftPortType=input  RightPortType=output  PseudoPeriodic=off  Frequencies=[]  VectorFormat=inherit  Unit=inherit  AffineConversion=off
  PS-Simulink Converter2 : nesl_utility/PS-Simulink Converter  PhysicalDomain=network_engine_domain  SubClassName=ps_output  LeftPortType=input  RightPortType=output  PseudoPeriodic=off  Frequencies=[]  VectorFormat=inherit  Unit=inherit  AffineConversion=off
  Voltage Sensor : fl_lib/Electrical/Electrical Sensors/Voltage Sensor
  + : PMIOPort  Side=Left
  - : PMIOPort  Port=2  Side=Left
  P : PMIOPort  Port=3  Side=Right
  N : PMIOPort  Port=4  Side=Right
  Bus Element Out : Outport  PortName=Meas  Element=SOC
  BusElementOut : Outport  PortName=Meas  Element=Vdc
  BusElementOut1 : Outport  PortName=Meas  Element=Ibatt
  BusElementOut2 : Outport  PortName=Meas  Element=Idc
  BusElementOut3 : Outport  PortName=Meas  Element=ILoad
  BusElementOut4 : Outport  PortName=Meas  Element=IDCDC
  BusElementOut5 : Outport  PortName=Meas  Element=UPSBrK
  wires:
  iPFC/1 -> Delay1/1
  Delay2/1 -> Low-Pass Filter (Discrete or Continuous)/1
  iChrg/1 -> BESS/3(iChrg)
  Delay1/1 -> BESS/1(iPFC)
  PS-Simulink Converter/1 -> Delay2/1
  BESS/1(Ibatt) -> BusElementOut1/1
  vPCC/1 -> BESS/4(vPCC)
  Brk/1 -> BusElementOut5/1, BESS/5(Brk)
  BESS/2(SOC) -> Bus Element Out/1
  Low-Pass Filter (Discrete or Continuous)/1 -> BESS/2(Vdc), BusElementOut/1
  PS-Simulink Converter1/1 -> Low-Pass Filter (Discrete or Continuous)1/1
  PS-Simulink Converter2/1 -> Low-Pass Filter (Discrete or Continuous)2/1
  Low-Pass Filter (Discrete or Continuous)2/1 -> BusElementOut3/1
  Low-Pass Filter (Discrete or Continuous)1/1 -> BusElementOut2/1
  BESS/3(IDCDC) -> BusElementOut4/1
  connections:
  Electrical Reference1/LConn1 -- N/RConn1 -- Voltage Sensor/RConn2 -- C1/RConn1 -- BESS/RConn1 -- -/RConn1
  PS-Simulink Converter/LConn1 -- Voltage Sensor/RConn1
  Voltage Sensor/LConn1 -- Current Sensor1/LConn1 -- Current Sensor/RConn2 -- BESS/LConn1 -- C1/LConn1
  PS-Simulink Converter1/LConn1 -- Current Sensor/RConn1
  P/RConn1 -- Current Sensor1/RConn2
  PS-Simulink Converter2/LConn1 -- Current Sensor1/RConn1
  Current Sensor/LConn1 -- +/RConn1
